simulink model "servo_test_system"  (Simulink 8.2)
settings: Solver=ode45  StartTime=0.0  StopTime=10.0  RelTol=1e-3
settings Model: Creator=David (non-admin)  LastModifiedBy=David (non-admin)
settings DataIOCC: SignalLoggingSaveFormat=Dataset
settings OptimizationCC: ExpressionDepthLimit=128
settings DebuggingCC: FcnCallInpInsideContextMsg=EnableAllAsError  StateNameClashWarn=none
settings GRTTargetCC: CombineOutputUpdateFcns=on  GRTInterface=off

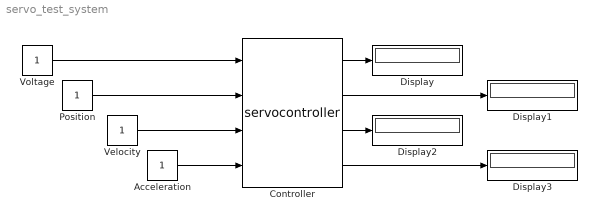
== system servo_test_system ==
  Acceleration : Constant
  Controller : M-S-Function  FunctionName=servocontroller
  Display{,1..3} (4 alike) : Display
  Position : Constant
  Velocity : Constant
  Voltage : Constant
  wires:
  Voltage/1 -> Controller/1
  Position/1 -> Controller/2
  Velocity/1 -> Controller/3
  Acceleration/1 -> Controller/4
  Controller/1 -> Display/1
  Controller/2 -> Display1/1
  Controller/3 -> Display2/1
  Controller/4 -> Display3/1
